simulink model "CorrectPV_2018a_102818"  (R2018a)
settings: Solver=VariableStepDiscrete  StartTime=0.0  StopTime=1  RelTol=1e-3
libraries: powerlib x38, simulink x4, re_lib x1
settings Model: Creator=mwkane  LastModifiedBy=mstruong

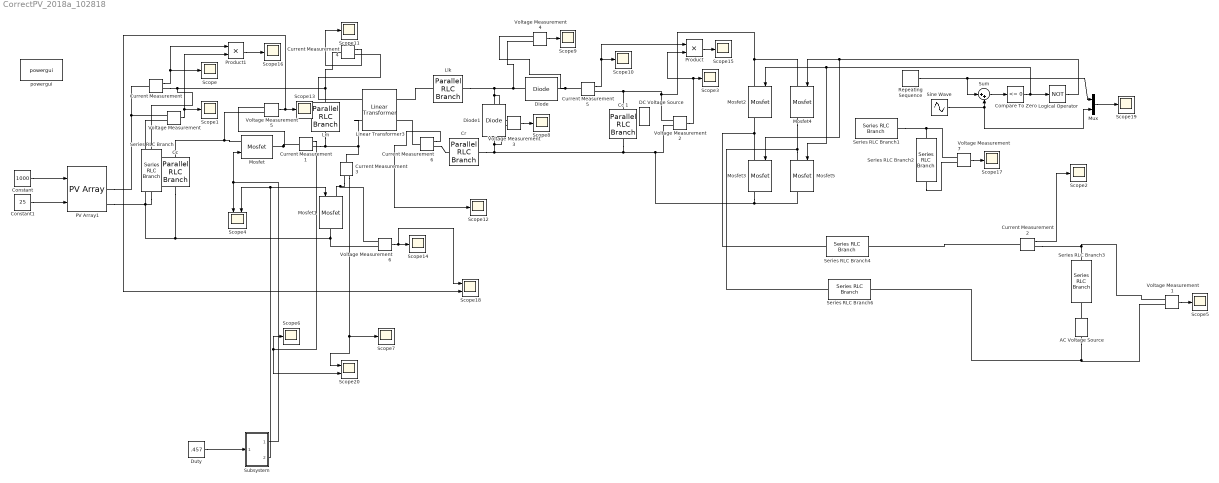
== system CorrectPV_2018a_102818 ==
  AC Voltage Source : powerlib/Electrical Sources/AC Voltage Source  Amplitude=220*sqrt(2)  Phase=0  Frequency=60  SampleTime=0  Measurements=None  BusType=swing  Pref=10e3  Qref=0  Qmin=-inf  Qmax=+inf
  "Cc " : powerlib/Elements/Parallel RLC Branch  LConnTagsString=a  RConnTagsString=__new0  BranchType=C  Resistance=1  Inductance=1e-3  SetiL0=off  InitialCurrent=0  Capacitance=2.2e-6  Setx0=off  InitialVoltage=0  Measurements=None
      settings: SourceProductName=Simscape Electrical
  Cc 1 : powerlib/Elements/Parallel RLC Branch  LConnTagsString=a  RConnTagsString=__new0  BranchType=C  Resistance=1  Inductance=1e-3  SetiL0=off  InitialCurrent=0  Capacitance=1e-3  Setx0=off  InitialVoltage=0  Measurements=None
      settings: SourceProductName=Simscape Electrical
  Compare To Zero : simulink/Logic and Bit Operations/Compare To Zero  relop=<=  OutDataTypeStr=boolean
  Constant : Constant  Value=1000
  Constant1 : Constant  Value=25
  Cr : powerlib/Elements/Parallel RLC Branch  LConnTagsString=a  RConnTagsString=__new0  BranchType=C  Resistance=1  Inductance=1e-3  SetiL0=off  InitialCurrent=0  Capacitance=2.4e-6  Setx0=off  InitialVoltage=0  Measurements=None
      settings: SourceProductName=Simscape Electrical
  Current Measurement{,1..6} (7 alike) : powerlib/Measurements/Current Measurement  PhasorSimulation=off  OutputType=Complex  PSBequivalent=0
      Current Measurement settings: SourceProductName=Simscape Electrical
      Current Measurement1 settings: SourceProductName=Simscape Electrical
      Current Measurement3 settings: SourceProductName=Simscape Electrical
      Current Measurement4 settings: SourceProductName=Simscape Electrical
      Current Measurement5 settings: SourceProductName=Simscape Electrical
      Current Measurement6 settings: SourceProductName=Simscape Electrical
  DC Voltage Source : powerlib/Electrical Sources/DC Voltage Source  Amplitude=350  Measurements=None
  Diode : powerlib/Power Electronics/Diode  Ron=0.001  Lon=0  Vf=.8  IC=0  UseSnubber=0  Rs=1e6  Cs=250e-9  Measurements=off
      settings: SourceProductName=Simscape Electrical
  Diode1 : powerlib/Power Electronics/Diode  Ron=0.001  Lon=0  Vf=.8  IC=0  UseSnubber=0  Rs=1e6  Cs=250e-9  Measurements=off
      settings: SourceProductName=Simscape Electrical
  Duty : Constant  Value=.457
  Linear Transformer3 : powerlib/Elements/Linear Transformer  UNITS=SI  NominalPower=[25 100e3]  winding1=[6.363961030678928 0 0]  winding2=[26.870057685088803 0 0]  ThreeWindings=off  winding3=[3.15e+05 3.969e+07 6316.9]  RmLm=[1e6 inf]  Measurements=None  DataType=on
      settings: SourceProductName=Simscape Electrical
  Llk : powerlib/Elements/Parallel RLC Branch  LConnTagsString=a  RConnTagsString=__new0  BranchType=L  Resistance=1  Inductance=2.6e-6  SetiL0=off  InitialCurrent=0  Capacitance=2.4e-6  Setx0=off  InitialVoltage=0  Measurements=None
      settings: SourceProductName=Simscape Electrical
  Lm : powerlib/Elements/Parallel RLC Branch  LConnTagsString=a  RConnTagsString=__new0  BranchType=L  Resistance=1  Inductance=20e-6  SetiL0=off  InitialCurrent=0  Capacitance=2.4e-6  Setx0=off  InitialVoltage=0  Measurements=None
      settings: SourceProductName=Simscape Electrical
  Logical Operator : Logic  Operator=NOT  AllPortsSameDT=off  OutDataTypeStr=boolean
  Mosfet : powerlib/Power Electronics/Mosfet  Ron=5.6e-3  Lon=0  Rd=0.01  Vfd=1.3  IC=0  Rs=1e5  Cs=inf  Measurements=off
      settings: SourceProductName=Simscape Electrical
  Mosfet1 : powerlib/Power Electronics/Mosfet  Ron=5.6e-3  Lon=0  Rd=0.01  Vfd=1.3  IC=0  Rs=1e6  Cs=inf  Measurements=off
      settings: SourceProductName=Simscape Electrical
  Mosfet{2..5} (4 alike) : powerlib/Power Electronics/Mosfet  Ron=0.1  Lon=0  Rd=0.01  Vfd=0  IC=0  Rs=1e5  Cs=inf  Measurements=on
  Mux : Mux  Inputs=2
  PV Array1 : re_lib/Solar/PV Array  Npar=1  Nser=2  PlotType=array @ 25 deg.C & specified irradiances  S_vec="[ 1000  500  100 ]"  Temp_C_vec="[ 45 25  ]"  ModuleName=User-defined  PlotWhenSelected=off  Pm=179.9805  Ncell=36  Voc=24.06  Isc=9.77  Vm=19.67  Im=9.15  beta_Voc_pc=-0.28  alpha_Isc_pc=+0.04  beta_Voc=-0.067368  alpha_Isc=0.003908  IL=9.8911  I0=1.3829e-11  nI=0.95443  Rsh=60.4787  Rs=0.18212  BAL=off  Tc=1e-6  Tfilter=5e-5
      settings: SourceProductName=Simscape Electrical
  Product : Product
  Product1 : Product
  Repeating Sequence : simulink/Sources/Repeating Sequence  rep_seq_t=[0 1/(4*(16000)) 3/(4*(16000)) 1/16000]  rep_seq_y=[0 1 -1 0]
  Scope{,1..3,5..17,19} (18 alike) : Scope
  Scope18 : Scope  NumInputPorts=2
  Scope20 : Scope  NumInputPorts=2
  Scope4 : Scope  NumInputPorts=2
  Series RLC Branch : powerlib/Elements/Series RLC Branch  LConnTagsString=__new0  RConnTagsString=__new0  BranchType=RC  Resistance=1e-6  Inductance=1e-3  SetiL0=off  InitialCurrent=0  Capacitance=1e-3  Setx0=off  InitialVoltage=0  Measurements=None
  Series RLC Branch1 : powerlib/Elements/Series RLC Branch  LConnTagsString=__new0  RConnTagsString=__new0  BranchType=RL  Resistance=1  Inductance=1e-3  SetiL0=off  InitialCurrent=0  Capacitance=1e-6  Setx0=off  InitialVoltage=0  Measurements=None
  Series RLC Branch2 : powerlib/Elements/Series RLC Branch  LConnTagsString=__new0  RConnTagsString=__new0  BranchType=RC  Resistance=1  Inductance=1e-3  SetiL0=off  InitialCurrent=0  Capacitance=1e-6  Setx0=off  InitialVoltage=0  Measurements=None
  Series RLC Branch3 : powerlib/Elements/Series RLC Branch  LConnTagsString=__new0  RConnTagsString=__new0  BranchType=RL  Resistance=10e-3  Inductance=2e-6  SetiL0=off  InitialCurrent=0  Capacitance=1e-6  Setx0=off  InitialVoltage=0  Measurements=None
  Series RLC Branch4 : powerlib/Elements/Series RLC Branch  LConnTagsString=__new0  RConnTagsString=__new0  BranchType=L  Resistance=1  Inductance=15e-3  SetiL0=off  InitialCurrent=0  Capacitance=15e-3  Setx0=off  InitialVoltage=0  Measurements=None
  Series RLC Branch6 : powerlib/Elements/Series RLC Branch  LConnTagsString=__new0  RConnTagsString=__new0  BranchType=L  Resistance=1  Inductance=15e-3  SetiL0=off  InitialCurrent=0  Capacitance=15e-3  Setx0=off  InitialVoltage=0  Measurements=None
  Sine Wave : Sin  Frequency=60*3.14*2  SampleTime=1e-6
  Subsystem : Subsystem
  Sum : Sum  Inputs=|++
  Voltage Measurement{,1..7} (8 alike) : powerlib/Measurements/Voltage Measurement  PhasorSimulation=off  OutputType=Complex  PSBequivalent=0
      Voltage Measurement settings: SourceProductName=Simscape Electrical
      Voltage Measurement2 settings: SourceProductName=Simscape Electrical
      Voltage Measurement3 settings: SourceProductName=Simscape Electrical
      Voltage Measurement4 settings: SourceProductName=Simscape Electrical
      Voltage Measurement5 settings: SourceProductName=Simscape Electrical
      Voltage Measurement6 settings: SourceProductName=Simscape Electrical
  powergui : powerlib/powergui  Priority=1  SimulationMode=Discrete  SampleTime=9e-8  frequency=60  Iterations=50  frequencyindice=0  Pbase=100e6  ErrMax=1e-4  UnitsV=kV  UnitsW=MW  buscounter=0  FunctionMessages=off  echomessages=off  EnableUseOfTLC=off  CurrentSourceSwitches=off  DisableSnubberDevices=off  DisableRonSwitches=off  DisableVfSwitches=off  DisplayEquations=off  SolverType=Tustin/Backward Euler (TBE)  Interpol=off  ExternalGateDelay=off  methode=off  Ts=100  x0status=blocks  SPID=on  SwTol=0  HookPort=off  RestoreLinks=warning  ResistiveCurrentMeasurement=off  Frange=[0:2:500]  Ylog=off  Xlog=on  ShowGrid=off  save=off  variable=ZData  structure=0  ZoomFFT=off  StartTime=0.0  cycles=1  DisplayStyle=1  fundamental=60  FreqAxis=off  MaxFrequency=1000  frequencyindicesteady=1  RmsSteady=1  display=off
  wires:
  Constant/1 -> PV Array1/1
  Constant1/1 -> PV Array1/2
  Current Measurement/1 -> Product1/1, Scope/1
  Voltage Measurement/1 -> Product1/2, Scope1/1
  Voltage Measurement2/1 -> Product/2, Scope3/1
  Subsystem/1(Out1) -> Mosfet/1, Scope4/1
  Subsystem/2(Out2) -> Mosfet1/1, Scope4/2
  Current Measurement5/1 -> Scope10/1, Product/1
  Product/1 -> Scope15/1
  Product1/1 -> Scope16/1
  Compare To Zero/1 -> Mosfet5/1, Mosfet2/1, Logical Operator/1
  Voltage Measurement7/1 -> Scope17/1
  Sum/1 -> Compare To Zero/1
  Logical Operator/1 -> Mosfet3/1, Mosfet4/1
  Sine Wave/1 -> Mux/2, Sum/2
  Repeating Sequence/1 -> Sum/1, Mux/1
  Mux/1 -> Scope19/1
  Current Measurement2/1 -> Scope2/1
  Voltage Measurement1/1 -> Scope5/1
  Current Measurement3/1 -> Scope20/1, Scope7/1
  Current Measurement1/1 -> Scope6/1, Scope20/2
  Voltage Measurement3/1 -> Scope8/1
  Voltage Measurement4/1 -> Scope9/1
  Current Measurement4/1 -> Scope11/1
  Current Measurement6/1 -> Scope12/1
  Voltage Measurement5/1 -> Scope18/2, Scope13/1
  Voltage Measurement6/1 -> Scope18/1, Scope14/1
  Duty/1 -> Subsystem/1(In1)
  connections:
  Voltage Measurement/LConn1 -- Current Measurement/LConn1 -- PV Array1/RConn1
  Voltage Measurement3/LConn1 -- Diode1/RConn1 -- Llk/RConn1 -- Voltage Measurement4/LConn2 -- Diode/LConn1
  PV Array1/RConn2 -- Mosfet1/RConn1 -- Voltage Measurement6/LConn2 -- "Cc "/RConn1 -- Series RLC Branch/RConn1 -- Voltage Measurement/LConn2
  Lm/RConn1 -- Linear Transformer3/LConn2 -- Current Measurement3/LConn1 -- Current Measurement1/RConn1
  Current Measurement5/LConn1 -- Voltage Measurement4/LConn1 -- Diode/RConn1
  Series RLC Branch1/RConn1 -- Voltage Measurement7/LConn1 -- Series RLC Branch2/LConn1
  Mosfet5/LConn1 -- Series RLC Branch6/LConn1 -- Mosfet4/RConn1
  Mosfet3/LConn1 -- Series RLC Branch4/LConn1 -- Mosfet2/RConn1
  Series RLC Branch3/LConn1 -- Voltage Measurement1/LConn1 -- Current Measurement2/RConn1
  AC Voltage Source/RConn1 -- Series RLC Branch3/RConn1
  Current Measurement3/RConn1 -- Voltage Measurement6/LConn1 -- Mosfet1/LConn1
  Voltage Measurement5/LConn2 -- Current Measurement1/LConn1 -- Mosfet/RConn1
  Linear Transformer3/LConn1 -- Current Measurement4/RConn1
  Current Measurement6/RConn1 -- Cr/LConn1
  Current Measurement4/LConn1 -- Series RLC Branch/LConn1 -- Current Measurement/RConn1 -- Lm/LConn1
  Voltage Measurement5/LConn1 -- "Cc "/LConn1 -- Mosfet/LConn1
  Llk/LConn1 -- Linear Transformer3/RConn1
  Current Measurement6/LConn1 -- Linear Transformer3/RConn2
  Mosfet3/RConn1 -- Cc 1/RConn1 -- Cr/RConn1 -- Voltage Measurement3/LConn2 -- Diode1/LConn1 -- Voltage Measurement2/LConn2 -- Mosfet5/RConn1
  AC Voltage Source/LConn1 -- Series RLC Branch6/RConn1 -- Voltage Measurement1/LConn2
  Current Measurement2/LConn1 -- Series RLC Branch4/RConn1
  Series RLC Branch2/RConn1 -- Voltage Measurement7/LConn2
  Mosfet2/LConn1 -- Cc 1/LConn1 -- Current Measurement5/RConn1 -- Voltage Measurement2/LConn1 -- Mosfet4/LConn1

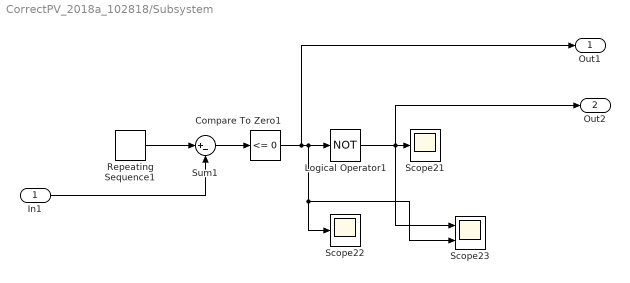
== system CorrectPV_2018a_102818/Subsystem ==
  In1 : Inport
  Compare To Zero1 : simulink/Logic and Bit Operations/Compare To Zero  relop=<=  OutDataTypeStr=boolean
  Logical Operator1 : Logic  Operator=NOT  AllPortsSameDT=off  OutDataTypeStr=boolean
  Repeating Sequence1 : simulink/Sources/Repeating Sequence  rep_seq_t=[0 1/50000]  rep_seq_y=[0 1]
  Scope21 : Scope
  Scope22 : Scope
  Scope23 : Scope  NumInputPorts=2
  Sum1 : Sum  Inputs=|+-
  Out1 : Outport
  Out2 : Outport  Port=2
  wires:
  Repeating Sequence1/1 -> Sum1/1
  Compare To Zero1/1 -> Out1/1, Scope23/2, Scope22/1, Logical Operator1/1
  In1/1 -> Sum1/2
  Logical Operator1/1 -> Out2/1, Scope23/1, Scope21/1
  Sum1/1 -> Compare To Zero1/1
